simulink library "cyclopsLib"  (R2020a)
settings: Solver=VariableStepAuto  StartTime=0.0  StopTime=10.0  RelTol=1e-3
values from neighbouring files (symbols this model uses):
  agc_delay_lag = 32    [rev0BB_setup.m]
  agc_detector_coef = ones(1,agc_detector_taps)./agc_detector_taps    [rev0BB_setup.m]
  agc_sat_low = -agcSaturation    (= -12)    [rev0BB_setup.m]
  agc_sat_up = agcSaturation    (= 12)    [rev0BB_setup.m]
  agcDesired = 0    [rev0BB_setup.m]
  agcExpDomain = agcSaturation    (= 12)    [rev0BB_setup.m]
  agcExpResolution = 2^-3    (= 0.125)    [rev0BB_setup.m]
  agcPwrAvgNum = 128    [rev0BB_setup.m]
  agcSettleThresh = 0.65    [rev0BB_setup.m]
  agcStep = 2^-8    (= 0.00390625)    [rev0BB_setup.m]
  atanDomain = 5    [rev0BB_setup.m]
  atanResolution = 2^-9    (= 0.001953125)    [rev0BB_setup.m]
  bitsPerSymbolHeader = log2(radixHeader)    [rev0BB_setup.m]
  bitsPerSymbolMax = log2(radixMax)    [rev0BB_setup.m]
  cefEarlyWarning = 256    [rev0BB_setup.m]
  cefLen = length(x_CEF)    [rev0BB_setup.m]
  coarseCFOAdaptDelay = 1    [rev0BB_setup.m]
  cr_i = 0.020    (= 0.02)    [rev0BB_setup.m]
  cr_i_preamp = 2^-9    (= 0.001953125)    [rev0BB_setup.m]
  cr_int1_sat_low = -cr_integrator1_saturation    (= -0.6)    [rev0BB_setup.m]
  cr_int1_sat_up = cr_integrator1_saturation    (= 0.6)    [rev0BB_setup.m]
  cr_integrator1_decay = 1    [rev0BB_setup.m]
  cr_integrator1_saturation = 0.6    [rev0BB_setup.m]
  cr_mult_pipeline = 1    [rev0BB_setup.m]
  cr_p = 0.015    [rev0BB_setup.m]
  cr_sat2_low = -cr_saturation2    (= -0.6)    [rev0BB_setup.m]
  cr_sat2_up = cr_saturation2    (= 0.6)    [rev0BB_setup.m]
  cr_smooth_num = (1/cr_smooth_samples).*ones(1, cr_smooth_samples)    [rev0BB_setup.m]
  D_32 = [ 1,  4,  8,  2, 16]    [golay.m]    (also in rev0BB_setup.m)
  dataLenSymbols = header_len_bytes*8/bitsPerSymbolHeader + frame_len_bytes*8/bitsPerSymbol    [rev0BB_setup.m]
  delayToOutputFromDataFSM = lmsEqDepth/2-1 + regular_pipeline*9 + cr_mult_pipeline*4    (= 31)    [rev0BB_setup.m]
  enableTRFreqCorrection = true    [rev0BB_setup.m]
  expDomain = 3.3    [rev0BB_setup.m]
  expResolution = 2^-5    (= 0.03125)    [rev0BB_setup.m]
  expTol = .1    (= 0.1)    [rev0BB_setup.m]
  forceSlowRxStrobed = false    [rev0BB_setup.m]
  frac_lut_domain_cr = 64    [rev0BB_setup.m]
  frac_lut_range_max_coarse_cfo = 127    [rev0BB_setup.m]
  frac_lut_range_max_cr = 127    [rev0BB_setup.m]
  frac_lut_range_min_coarse_cfo = -frac_lut_range_max_coarse_cfo    (= -127)    [rev0BB_setup.m]
  frac_lut_range_min_cr = -frac_lut_range_max_cr    (= -127)    [rev0BB_setup.m]
  frac_lut_table_breaks_coarse_cfo = -frac_lut_domain_coarse_cfo:frac_lut_res_coarse_cfo:(frac_lut_domain_coarse_cfo-1)    [rev0BB_setup.m]
  frac_lut_table_breaks_cr = -frac_lut_domain_cr:frac_lut_res_cr:(frac_lut_domain_cr-1)    [rev0BB_setup.m]
  frac_lut_table_data_coarse_cfo = 1./frac_lut_table_breaks_coarse_cfo    [rev0BB_setup.m]
  frac_lut_table_data_cr = 1./frac_lut_table_breaks_cr    [rev0BB_setup.m]
  golay_type = 32    [rev0BB_setup.m]
  header_len_bytes = 8    [rev0BB_setup.m]
  lmsEqDepth = 38    [rev0BB_setup.m]
  lmsStep_init = 0.012    [rev0BB_setup.m]
  lmsStep_meta = (lmsStep_final - lmsStep_init)/cefLen    [rev0BB_setup.m]
  lnDomain = 16    [rev0BB_setup.m]
  lnResolution = 2^-3    (= 0.125)    [rev0BB_setup.m]
  minSTFPeaks = 3    [rev0BB_setup.m]
  mod_scheme_len_bytes = 1    [rev0BB_setup.m]
  modBPS = [1, 2, 4]    [rev0BB_setup.m]
  modKeys = [0, 1, 2]    [rev0BB_setup.m]
  mult_pipeline = 1    [rev0BB_setup.m]
  overSample = 4    [berCurve.m]    (also in rev0BB_setup.m)
  overSamplePer = 1/overSampleFreq    (= 1.25e-08)    [rev0BB_setup.m]
  qam16_demod_scale_factor = qam16_hdl_distance/qam16_power_normalized_distance    [rev0BB_setup.m]
  rcRxFilt = rcSqrtFilt    [rev0BB_setup.m]
  rcTxFilt = rcSqrtFilt    [rev0BB_setup.m]
  regular_pipeline = 1    [rev0BB_setup.m]
  rx_gain = 1    [rev0BB_setup.m]
  rx_gain_i = 1    [rev0BB_setup.m]
  rx_gain_q = 1    [rev0BB_setup.m]
  RxFeedbackPipelining = 128*3    (= 384)    [rev0BB_setup.m]
  stfLen = length(x_STF)    [rev0BB_setup.m]
  timing_differentiator_grpDelay_roundUp = ceil((timing_differentiator_len)/2)    [rev0BB_setup.m]
  timing_integrator1_decay = 0.999    [rev0BB_setup.m]
  timing_p = -1/2^2 -1/2^3    (= -0.375)    [rev0BB_setup.m]
  timing_tolerance = 4    [rev0BB_setup.m]
  timingRecoveryDoneSamplesEarly = 1    [rev0BB_setup.m]
  timingRecoveryDoneSamplesEarlyExtraDelay = -timingRecoveryDoneSamplesEarly+1    (= 0)    [rev0BB_setup.m]
  tr_int1_sat_low = -timing_integrate1_saturate    (= -0.0025)    [rev0BB_setup.m]
  tr_int1_sat_up = timing_integrate1_saturate    (= 0.0025)    [rev0BB_setup.m]
  tr_sat2_low = -timing_saturate2    (= -0.005)    [rev0BB_setup.m]
  tr_sat2_up = timing_saturate2    (= 0.005)    [rev0BB_setup.m]
  trigger = 0.40    (= 0.4)    [rev0BB_setup.m]
  trigger_tolerance = 0.35    [rev0BB_setup.m]
  W_32 = [-1,  1, -1,  1, -1]    [golay.m]    (also in rev0BB_setup.m)
  x_STFRepCount = nSpectrum_STFRepCount_short    (= 60)    [rev0BB_setup.m]
undefined symbols (not defined in the file or in its folder): agc_on, cr_integrator2_saturation, Fast_Rx_Partition, Fast_Slim_Rx_Partition, Feedback_Pipeline, freeze_en_agc, freeze_en_cr_int1, freeze_en_cr_int2, freeze_en_cr_phase, freeze_en_tr_int1, freeze_en_tr_int2, freeze_en_tr_phase, freeze_on_cef_done, freeze_on_stf_done, freeze_on_valid, i, post_cr_i_offset, post_cr_q_offset, rx_offset_correction_i, rx_offset_correction_q, Slow_Rx_Partition, timing_i, timing_i_pre_scale
libraries: simulink x62, helperLib x48, golayLib x15, commdigbbndpm3 x8, commdigbbndam3 x4, commfilt2 x3, hdlsllib x2, dspfdesign x1, simulink_need_slupdate x1, dspsigops x1, dsphdlsigops x1, $bdroot x1
(part 4 of 5)

== system cyclopsLib/cyclops_rx_combined/slow_rx_encapsulated/slow_rx/slow_rx_baseband_outer/slow_rx_baseband_enabled/slow_rx_baseband/header_parse_ack_decision ==
  note: min frame length of 2 symbols
  crc_decision : Inport
  data : Inport  Port=2
  valid : Inport  Port=3
  Data Type Conversion{4..7} (4 alike) : DataTypeConversion  Commented=on
  Delay2 : Delay  DelayLength=1  InitialCondition=0
  Display2 : Display  Commented=on
  Terminator{1..11} (11 alike) : Terminator
  Vector Concatenate1 : Concatenate  Commented=on  NumInputs=4
  header_parse_ack : Stateflow chart  TreatAsAtomicUnit=on
  majority : Subsystem
  mod_type_valid : Outport  VectorParamsAs1DForOutWhenUnconnected=off
  mod_type : Outport  Port=2  VectorParamsAs1DForOutWhenUnconnected=off
  payload_early : Outport  Port=3  VectorParamsAs1DForOutWhenUnconnected=off
  payload : Outport  Port=4  VectorParamsAs1DForOutWhenUnconnected=off
  wires:
  majority/1(Out1) -> mod_type/1
  header_parse_ack/7(mod_type) -> majority/1(In1)
  Data Type Conversion4/1 -> Vector Concatenate1/1
  Data Type Conversion5/1 -> Vector Concatenate1/2
  Data Type Conversion7/1 -> Vector Concatenate1/4
  Data Type Conversion6/1 -> Vector Concatenate1/3
  header_parse_ack/8(type) -> Terminator9/1, Data Type Conversion4/1
  header_parse_ack/6(done_parsing) -> Terminator7/1
  valid/1 -> header_parse_ack/2(valid)
  header_parse_ack/4(dst_valid) -> Terminator5/1
  header_parse_ack/5(len_valid) -> Terminator6/1
  header_parse_ack/3(src_valid) -> Terminator4/1
  data/1 -> header_parse_ack/1(data)
  crc_decision/1 -> Delay2/1
  header_parse_ack/9(src) -> Terminator8/1, Data Type Conversion5/1
  Delay2/1 -> header_parse_ack/3(rst)
  Vector Concatenate1/1 -> Display2/1
  header_parse_ack/10(dst) -> Data Type Conversion6/1, Terminator2/1
  header_parse_ack/11(len) -> Terminator1/1, Data Type Conversion7/1
  header_parse_ack/2(type_valid) -> Terminator3/1
  header_parse_ack/1(mod_type_valid) -> mod_type_valid/1
  header_parse_ack/13(payload_early) -> payload_early/1
  header_parse_ack/12(payload) -> payload/1
  header_parse_ack/14(net_id_valid) -> Terminator10/1
  header_parse_ack/15(net_id) -> Terminator11/1

== system cyclopsLib/cyclops_rx_combined/slow_rx_encapsulated/slow_rx/slow_rx_baseband_outer/slow_rx_baseband_enabled/slow_rx_baseband/mod_data_buffer ==
  data : Inport
  header : Inport  Port=2
  payload : Inport  Port=3
  last_in : Inport  Port=4
  bitsPerSymbolPayload : Inport  Port=5
  rst : Inport  Port=6
  header_parse_and_buffer : Stateflow chart  TreatAsAtomicUnit=on
  packed_data : Outport  VectorParamsAs1DForOutWhenUnconnected=off
  valid : Outport  Port=2  VectorParamsAs1DForOutWhenUnconnected=off
  last_out : Outport  Port=3  VectorParamsAs1DForOutWhenUnconnected=off
  decoding : Outport  Port=4  VectorParamsAs1DForOutWhenUnconnected=off
  err : Outport  Port=5  VectorParamsAs1DForOutWhenUnconnected=off
  wires:
  data/1 -> header_parse_and_buffer/4(data)
  header/1 -> header_parse_and_buffer/2(header)
  header_parse_and_buffer/2(packed_data) -> packed_data/1
  header_parse_and_buffer/3(valid) -> valid/1
  header_parse_and_buffer/1(last_out) -> last_out/1
  payload/1 -> header_parse_and_buffer/5(payload)
  last_in/1 -> header_parse_and_buffer/1(last_in)
  bitsPerSymbolPayload/1 -> header_parse_and_buffer/3(bitsPerSymbolMod)
  rst/1 -> header_parse_and_buffer/6(rst)
  header_parse_and_buffer/4(decoding) -> decoding/1
  header_parse_and_buffer/5(err) -> err/1

== system cyclopsLib/cyclops_rx_combined/slow_rx_encapsulated/slow_rx/slow_rx_baseband_outer/slow_rx_baseband_enabled/slow_rx_baseband/nco ==
  incr : Inport
  Data Type Conversion3 : DataTypeConversion  OutDataTypeStr=int32
  Display : Display  Commented=on
  Display1 : Display  Commented=on
  NCO : dspsigops/NCO  AccIncSrc=Input port  AccInc=100  PhaseOffsetSrc=Specify via dialog  PhaseOffset=0  AccumWL=16  HasDither=off  DitherWL=4  PNgeneratorLength=19  HasPhaseQuantizer=on  TableDepth=12  HasOutputPhaseError=off  Formula=Complex exponential  DataType=single  OutputWL=18  OutputFL=13  CompMethod=Table lookup (no interpolation)  SampleTime=1  SamplesPerFrame=1  OutputFrames=off
      settings: SourceProductBaseCode=DS
  NCO HDL Optimized : dsphdlsigops/NCO HDL Optimized  Commented=on  PhaseIncrementSource=Input port  PhaseIncrement=100  PhaseOffsetSource=Property  PhaseOffset=0  DitherSource=None  NumDitherBits=4  SamplesPerFrame=1  LUTCompress=on  ResetAction=off  Waveform=Complex exponential  PhasePort=on  SimulateUsing=Code generation  AccumulatorWL=22  PhaseQuantization=on  NumQuantizerAccumulatorBits=20  OutputDataType=Binary point scaling  OutputWL=18  OutputFL=13
      settings: SourceProductBaseCode=DS
  Signal Specification : SignalSpecification  Commented=on  Dimensions=1
  Terminator1 : Terminator  Commented=on
  nco_phase : Scope  Commented=on
  incr_int : Outport  VectorParamsAs1DForOutWhenUnconnected=off
  complex_sin : Outport  Port=2  VectorParamsAs1DForOutWhenUnconnected=off
  wires:
  Data Type Conversion3/1 -> Display1/1, NCO/1, incr_int/1, Signal Specification/1
  NCO/1 -> complex_sin/1
  incr/1 -> Display/1, Data Type Conversion3/1
  NCO HDL Optimized/3 -> Terminator1/1
  NCO HDL Optimized/2 -> nco_phase/1

== system cyclopsLib/cyclops_rx_combined/slow_rx_encapsulated/slow_rx/slow_rx_baseband_outer/slow_rx_baseband_enabled/slow_rx_baseband/preamble_data_ctrl ==
  stfStart : Inport
  cefStart : Inport  Port=2
  Data Type Conversion : DataTypeConversion  OutDataTypeStr=boolean
  Terminator : Terminator
  Terminator1 : Terminator
  cef_eq_fsm : Stateflow chart  TreatAsAtomicUnit=on
  data_control : Stateflow chart  TreatAsAtomicUnit=on
  dataValid : Outport  VectorParamsAs1DForOutWhenUnconnected=off
  cefSymb : Outport  Port=2  VectorParamsAs1DForOutWhenUnconnected=off
  dataLast : Outport  Port=3  VectorParamsAs1DForOutWhenUnconnected=off
  err : Outport  Port=4  VectorParamsAs1DForOutWhenUnconnected=off
  stf : Outport  Port=5  VectorParamsAs1DForOutWhenUnconnected=off
  cef : Outport  Port=6  VectorParamsAs1DForOutWhenUnconnected=off
  cefCount : Outport  Port=7  VectorParamsAs1DForOutWhenUnconnected=off
  preamble_done : Outport  Port=8  VectorParamsAs1DForOutWhenUnconnected=off
  cefEarly : Outport  Port=9  VectorParamsAs1DForOutWhenUnconnected=off
  ack : Outport  Port=10  VectorParamsAs1DForOutWhenUnconnected=off
  ack_done : Outport  Port=11  VectorParamsAs1DForOutWhenUnconnected=off
  ack_dst : Outport  Port=12  VectorParamsAs1DForOutWhenUnconnected=off
  ack_trigger : Outport  Port=13  VectorParamsAs1DForOutWhenUnconnected=off
  dataLast_early : Outport  Port=14  VectorParamsAs1DForOutWhenUnconnected=off
  wires:
  data_control/3(earlyLast) -> dataLast_early/1
  cefStart/1 -> cef_eq_fsm/2(cef_start)
  stfStart/1 -> cef_eq_fsm/1(stf_start)
  cef_eq_fsm/1(data) -> Data Type Conversion/1
  cef_eq_fsm/3(cefSymb) -> cefSymb/1
  cef_eq_fsm/6(cefCount) -> cefCount/1
  cef_eq_fsm/7(cef_early) -> cefEarly/1
  data_control/1(valid) -> dataValid/1
  cef_eq_fsm/2(err) -> err/1
  cef_eq_fsm/4(stf) -> stf/1
  cef_eq_fsm/5(cef) -> cef/1
  data_control/2(last) -> dataLast/1
  cef_eq_fsm/8(waiting) -> Terminator/1
  cef_eq_fsm/10(ack) -> ack/1
  cef_eq_fsm/9(ack_done) -> ack_done/1
  cef_eq_fsm/11(ack_dst) -> ack_dst/1
  cef_eq_fsm/12(ack_count) -> Terminator1/1
  cef_eq_fsm/13(ack_trigger) -> ack_trigger/1
  Data Type Conversion/1 -> preamble_done/1, data_control/1(preamble_done)

== system cyclopsLib/cyclops_rx_combined/slow_rx_encapsulated/slow_rx/slow_rx_baseband_outer/slow_rx_baseband_enabled/slow_rx_baseband/CoarseCFO_est/atan ==
  note: 5 delays
  note: Special case for undefined ouput of atan2.
      | To produce an unbiased ouput, this should be 0.
  imag_y : Inport
  real_x : Inport  Port=2
  Compare To Constant2 : simulink/Logic and Bit Operations/Compare To Constant  relop=>=  const=0  OutDataTypeStr=boolean
  Compare To Constant3 : simulink/Logic and Bit Operations/Compare To Constant  relop===  const=0  OutDataTypeStr=boolean
  Compare To Constant4 : simulink/Logic and Bit Operations/Compare To Constant  relop===  const=0  OutDataTypeStr=boolean
  Constant2 : Constant  Value=0  OutDataTypeStr=Inherit: Inherit via back propagation  SampleTime=-1
  Constant3 : Constant  Value=-pi/2  OutDataTypeStr=Inherit: Inherit via back propagation  SampleTime=-1
  Constant4 : Constant  Value=pi/2  OutDataTypeStr=Inherit: Inherit via back propagation  SampleTime=-1
  Logical Operator : Logic  AllPortsSameDT=off  OutDataTypeStr=boolean
  Logical Operator1 : Logic  AllPortsSameDT=off  OutDataTypeStr=boolean
  Switch3 : Switch  Criteria=u2 ~= 0  OutDataTypeStr=Inherit: Inherit via back propagation
  Switch4 : Switch  Criteria=u2 ~= 0  OutDataTypeStr=Inherit: Inherit via back propagation
  Switch5 : Switch  Criteria=u2 ~= 0  OutDataTypeStr=Inherit: Inherit via back propagation
  bound_atan : Subsystem  AncestorBlock=helperLib/bound_atan
  inv : Subsystem
  mult_delay_match : Delay  DelayLength=cr_mult_pipeline*2+regular_pipeline*2
  pipeline_delay{,1..3} (4 alike) : Delay  DelayLength=regular_pipeline
  pipeline_delay_match2 : Delay  DelayLength=cr_mult_pipeline*5+regular_pipeline*7
  pipeline_delay_match3 : Delay  DelayLength=cr_mult_pipeline*5+regular_pipeline*7
  pipeline_delay_match4 : Delay  DelayLength=cr_mult_pipeline*5+regular_pipeline*7
  pipelined_mult : helperLib/pipelined_mult  d=cr_mult_pipeline
  Out1 : Outport  VectorParamsAs1DForOutWhenUnconnected=off
  wires:
  pipeline_delay1/1 -> bound_atan/1(In1)
  imag_y/1 -> Compare To Constant4/1, Compare To Constant2/1, mult_delay_match/1
  mult_delay_match/1 -> pipeline_delay2/1
  bound_atan/1(Out1) -> pipeline_delay/1
  pipelined_mult/1 -> pipeline_delay1/1
  pipeline_delay2/1 -> pipelined_mult/1
  pipeline_delay3/1 -> pipelined_mult/2
  Compare To Constant4/1 -> Logical Operator/1
  Logical Operator/1 -> pipeline_delay_match2/1
  pipeline_delay_match2/1 -> Switch3/2
  real_x/1 -> inv/1(In), Compare To Constant3/1
  inv/1(Out) -> pipeline_delay3/1
  Switch4/1 -> Switch5/3
  Constant3/1 -> Switch4/1
  Constant4/1 -> Switch5/1
  Switch5/1 -> Switch3/3
  Constant2/1 -> Switch3/1
  Compare To Constant3/1 -> Logical Operator1/2, pipeline_delay_match4/1, Logical Operator/2
  Logical Operator1/1 -> pipeline_delay_match3/1
  pipeline_delay_match3/1 -> Switch5/2
  pipeline_delay_match4/1 -> Switch4/2
  Compare To Constant2/1 -> Logical Operator1/1
  pipeline_delay/1 -> Switch4/3
  Switch3/1 -> Out1/1

== system cyclopsLib/cyclops_rx_combined/slow_rx_encapsulated/slow_rx/slow_rx_baseband_outer/slow_rx_baseband_enabled/slow_rx_baseband/CoarseCFO_est/complex_mult_pipelined1 ==
  In1 : Inport
  In2 : Inport  Port=2
  Add1 : Sum  OutDataTypeStr=Inherit: Same as first input
  Add2 : Sum  OutDataTypeStr=Inherit: Same as first input
  Complex to Real-Imag3 : ComplexToRealImag
  Complex to Real-Imag4 : ComplexToRealImag
  Real-Imag to Complex2 : RealImagToComplex
  mult_delay_match3 : Delay  DelayLength=cr_mult_pipeline
  mult_delay_match4 : Delay  DelayLength=cr_mult_pipeline
  mult_delay_match5 : Delay  DelayLength=cr_mult_pipeline
  pipeline_delay{1..3,6} (4 alike) : Delay  DelayLength=regular_pipeline
  pipelined_gain : helperLib/pipelined_gain  g=-1  d=cr_mult_pipeline
  pipelined_mult{,1..3} (4 alike) : helperLib/pipelined_mult  d=cr_mult_pipeline
  Out1 : Outport  VectorParamsAs1DForOutWhenUnconnected=off
  wires:
  pipelined_gain/1 -> Add1/2
  pipelined_mult3/1 -> mult_delay_match5/1
  pipelined_mult2/1 -> mult_delay_match4/1
  pipelined_mult1/1 -> pipelined_gain/1
  pipelined_mult/1 -> mult_delay_match3/1
  Complex to Real-Imag4/1 -> pipelined_mult/2, pipelined_mult3/2
  Complex to Real-Imag3/2 -> pipelined_mult1/1, pipelined_mult3/1
  Complex to Real-Imag4/2 -> pipelined_mult2/2, pipelined_mult1/2
  Complex to Real-Imag3/1 -> pipelined_mult2/1, pipelined_mult/1
  pipeline_delay3/1 -> Complex to Real-Imag4/1
  pipeline_delay2/1 -> Complex to Real-Imag3/1
  Add2/1 -> pipeline_delay6/1
  Add1/1 -> pipeline_delay1/1
  In1/1 -> pipeline_delay2/1
  mult_delay_match5/1 -> Add2/2
  pipeline_delay1/1 -> Real-Imag to Complex2/1
  In2/1 -> pipeline_delay3/1
  pipeline_delay6/1 -> Real-Imag to Complex2/2
  Real-Imag to Complex2/1 -> Out1/1
  mult_delay_match3/1 -> Add1/1
  mult_delay_match4/1 -> Add2/1

== system cyclopsLib/cyclops_rx_combined/slow_rx_encapsulated/slow_rx/slow_rx_baseband_outer/slow_rx_baseband_enabled/slow_rx_baseband/EQ/lms ==
  in : Inport
  expected : Inport  Port=2
  reset : Inport  Port=3
  adapt : Inport  Port=4
  step : Inport  Port=5
  Constant : Constant  Value=complex(cat(1,zeros(lmsEqDepth/2-1,1), [1], zeros(lmsEqDepth/2,1)))  OutDataTypeStr=Inherit: Inherit via back propagation  SampleTime=-1
  Data Type Conversion : DataTypeConversion  OutDataTypeStr=single
  Data Type Conversion1 : DataTypeConversion  OutDataTypeStr=single
  Data Type Conversion2 : DataTypeConversion  OutDataTypeStr=single
  Delay : Delay  DelayLength=1
  Delay3 : Delay  DelayLength=lmsEqDepth/2-1  InitialCondition=0
  Discrete FIR Filter : DiscreteFir  CoefSource=Input port  FilterStructure=Direct form transposed  OutDataTypeStr=Inherit: Same as input
      settings: InputPortMap=u0,u1
  Display : Display  Commented=on
  Product : Product  OutDataTypeStr=Inherit: Same as first input
  Product1 : Product  OutDataTypeStr=Inherit: Same as first input
  Sum : Sum  Inputs=|+-  OutDataTypeStr=Inherit: Same as first input
  Sum1 : Sum  Inputs=|++  OutDataTypeStr=Inherit: Same as first input
  Switch : Switch  Criteria=u2 > Threshold
  Switch1 : Switch  Criteria=u2 > Threshold
  Tapped Delay : simulink/Discrete/Tapped Delay  vinit=0.0  samptime=-1  NumDelays=lmsEqDepth-1  DelayOrder=Newest  includeCurrent=off
  Unit Delay Resettable : simulink_need_slupdate/Unit Delay Resettable  Commented=on  vinit=complex(cat(1,zeros(lmsEqDepth/2-1,1), [1], zeros(lmsEqDepth/2,1)))  tsamp=-1
      settings: SourceProductBaseCode=SL
  Vector Concatenate : Concatenate
  complex_conj : helperLib/complex_conj  SystemSampleTime=-1  Latency=0  AutoFrameSizeCalculation=off
  pipeline_delay{1,3..6} (5 alike) : Delay  DelayLength=regular_pipeline
  out : Outport  VectorParamsAs1DForOutWhenUnconnected=off
  err : Outport  Port=2  VectorParamsAs1DForOutWhenUnconnected=off
  wires:
  Tapped Delay/1 -> Vector Concatenate/2
  Data Type Conversion2/1 -> pipeline_delay6/1
  complex_conj/1 -> Tapped Delay/1, Vector Concatenate/1
  Sum1/1 -> Switch/1
  Data Type Conversion1/1 -> pipeline_delay1/1
  Data Type Conversion/1 -> Delay3/1
  step/1 -> pipeline_delay3/1
  Delay3/1 -> pipeline_delay4/1
  adapt/1 -> Switch/2
  pipeline_delay1/1 -> complex_conj/1, Discrete FIR Filter/1
  Delay/1 -> Sum1/1, Display/1, Switch/3, Discrete FIR Filter/2
  reset/1 -> Switch1/2
  expected/1 -> Data Type Conversion/1
  in/1 -> Data Type Conversion1/1
  pipeline_delay5/1 -> err/1
  pipeline_delay6/1 -> out/1
  Sum/1 -> Product/1, pipeline_delay5/1
  pipeline_delay3/1 -> Product/2
  Product/1 -> Product1/1
  Vector Concatenate/1 -> Product1/2
  pipeline_delay4/1 -> Sum/1
  Discrete FIR Filter/1 -> Sum/2, Data Type Conversion2/1
  Product1/1 -> Sum1/2
  Switch/1 -> Switch1/3
  Switch1/1 -> Delay/1
  Constant/1 -> Switch1/1

== system cyclopsLib/cyclops_rx_combined/slow_rx_encapsulated/slow_rx/slow_rx_baseband_outer/slow_rx_baseband_enabled/slow_rx_baseband/FineCarrierRecovery/Est_Phase ==
  In1 : Inport
  ModMode : Inport  Port=2
  Atan2 : Trigonometry  Operator=atan2
  Complex to Real-Imag : ComplexToRealImag
  Complex to Real-Imag1 : ComplexToRealImag
  Data Type Conversion : DataTypeConversion  OutDataTypeStr=single
  Gain : Gain  Gain=-1  OutDataTypeStr=Inherit: Same as input
  Real-Imag to Complex1 : RealImagToComplex
  atan2 : Subsystem  Commented=on  AncestorBlock=helperLib/atan2
  complex_mult_pipelined1 : Subsystem  AncestorBlock=helperLib/complex_mult_pipelined
  find_nearest : Subsystem
  mult_delay5 : Delay  DelayLength=cr_mult_pipeline
  mult_delay_match : Delay  DelayLength=cr_mult_pipeline
  mult_delay_match2 : Delay  DelayLength=cr_mult_pipeline
  pipeline_delay2 : Delay  DelayLength=regular_pipeline
  phase_offset : Outport  VectorParamsAs1DForOutWhenUnconnected=off
  wires:
  mult_delay_match2/1 -> complex_mult_pipelined1/1(In1)
  find_nearest/1(Out1) -> mult_delay_match2/1
  Data Type Conversion/1 -> Complex to Real-Imag/1, find_nearest/1(In1)
  Atan2/1 -> pipeline_delay2/1
  Complex to Real-Imag1/2 -> Atan2/1
  Complex to Real-Imag1/1 -> Atan2/2
  pipeline_delay2/1 -> phase_offset/1
  Gain/1 -> Real-Imag to Complex1/2
  mult_delay_match/1 -> Real-Imag to Complex1/1
  Real-Imag to Complex1/1 -> complex_mult_pipelined1/2(In2)
  Complex to Real-Imag/2 -> mult_delay5/1
  Complex to Real-Imag/1 -> mult_delay_match/1
  In1/1 -> Data Type Conversion/1
  mult_delay5/1 -> Gain/1
  complex_mult_pipelined1/1(Out1) -> Complex to Real-Imag1/1
  ModMode/1 -> find_nearest/2(ModMode)

== system cyclopsLib/cyclops_rx_combined/slow_rx_encapsulated/slow_rx/slow_rx_baseband_outer/slow_rx_baseband_enabled/slow_rx_baseband/FineCarrierRecovery/PostCR_IQ_Offset_Correct ==
  In : Inport
  post_cr_i_offset : Inport  Port=2
  post_cr_q_offset : Inport  Port=3
  Add : Sum  OutDataTypeStr=Inherit: Same as first input
  Add1 : Sum  OutDataTypeStr=Inherit: Same as first input
  Complex to Real-Imag1 : ComplexToRealImag
  Real-Imag to Complex1 : RealImagToComplex
  pipeline_delay : Delay  DelayLength=regular_pipeline
  pipeline_delay1 : Delay  DelayLength=regular_pipeline
  Out : Outport  VectorParamsAs1DForOutWhenUnconnected=off
  wires:
  Real-Imag to Complex1/1 -> Out/1
  Add/1 -> pipeline_delay/1
  Complex to Real-Imag1/2 -> Add1/1
  Complex to Real-Imag1/1 -> Add/1
  Add1/1 -> pipeline_delay1/1
  In/1 -> Complex to Real-Imag1/1
  post_cr_q_offset/1 -> Add1/2
  post_cr_i_offset/1 -> Add/2
  pipeline_delay/1 -> Real-Imag to Complex1/1
  pipeline_delay1/1 -> Real-Imag to Complex1/2

== system cyclopsLib/cyclops_rx_combined/slow_rx_encapsulated/slow_rx/slow_rx_baseband_outer/slow_rx_baseband_enabled/slow_rx_baseband/FineCarrierRecovery/complex_mult_pipelined ==
  In1 : Inport
  In2 : Inport  Port=2
  Add1 : Sum  OutDataTypeStr=Inherit: Same as first input
  Add2 : Sum  OutDataTypeStr=Inherit: Same as first input
  Complex to Real-Imag3 : ComplexToRealImag
  Complex to Real-Imag4 : ComplexToRealImag
  Real-Imag to Complex2 : RealImagToComplex
  mult_delay_match3 : Delay  DelayLength=cr_mult_pipeline
  mult_delay_match4 : Delay  DelayLength=cr_mult_pipeline
  mult_delay_match5 : Delay  DelayLength=cr_mult_pipeline
  pipeline_delay{1..3,6} (4 alike) : Delay  DelayLength=regular_pipeline
  pipelined_gain : helperLib/pipelined_gain  g=-1  d=cr_mult_pipeline
  pipelined_mult{,1..3} (4 alike) : helperLib/pipelined_mult  d=cr_mult_pipeline
  Out1 : Outport  VectorParamsAs1DForOutWhenUnconnected=off
  wires:
  pipelined_gain/1 -> Add1/2
  pipelined_mult3/1 -> mult_delay_match5/1
  pipelined_mult2/1 -> mult_delay_match4/1
  pipelined_mult1/1 -> pipelined_gain/1
  pipelined_mult/1 -> mult_delay_match3/1
  Complex to Real-Imag4/1 -> pipelined_mult/2, pipelined_mult3/2
  Complex to Real-Imag3/2 -> pipelined_mult1/1, pipelined_mult3/1
  Complex to Real-Imag4/2 -> pipelined_mult2/2, pipelined_mult1/2
  Complex to Real-Imag3/1 -> pipelined_mult2/1, pipelined_mult/1
  pipeline_delay3/1 -> Complex to Real-Imag4/1
  pipeline_delay2/1 -> Complex to Real-Imag3/1
  Add2/1 -> pipeline_delay6/1
  Add1/1 -> pipeline_delay1/1
  In1/1 -> pipeline_delay2/1
  mult_delay_match5/1 -> Add2/2
  pipeline_delay1/1 -> Real-Imag to Complex2/1
  In2/1 -> pipeline_delay3/1
  pipeline_delay6/1 -> Real-Imag to Complex2/2
  Real-Imag to Complex2/1 -> Out1/1
  mult_delay_match3/1 -> Add1/1
  mult_delay_match4/1 -> Add2/1

== system cyclopsLib/cyclops_rx_combined/slow_rx_encapsulated/slow_rx/slow_rx_baseband_outer/slow_rx_baseband_enabled/slow_rx_baseband/FineCarrierRecovery/overflow_protect ==
  note: Synthesizer
  note: This fixes overflow problem with LUT.  This keeps the
      | signal from -pi to pi plus some hystoresis if the LUT's
      | domain is slightly larger than -pi to pi
  In1 : Inport
  Compare To Constant2 : simulink/Logic and Bit Operations/Compare To Constant  relop=>=  const=expDomain-expTol  OutDataTypeStr=boolean
  Compare To Constant3 : simulink/Logic and Bit Operations/Compare To Constant  relop=<=  const=-expDomain+expTol  OutDataTypeStr=boolean
  Constant1 : Constant  Value=2*pi  OutDataTypeStr=Inherit: Inherit via back propagation  SampleTime=-1
  Constant2 : Constant  Value=0  OutDataTypeStr=Inherit: Inherit via back propagation  SampleTime=-1
  Sum4 : Sum  Inputs=|+-  OutDataTypeStr=Inherit: Same as first input
  Sum5 : Sum  Inputs=|++  OutDataTypeStr=Inherit: Same as first input
  Switch : Switch  Criteria=u2 ~= 0  OutDataTypeStr=Inherit: Inherit via back propagation
  Switch1 : Switch  Criteria=u2 ~= 0  OutDataTypeStr=Inherit: Inherit via back propagation
  Out1 : Outport  VectorParamsAs1DForOutWhenUnconnected=off
  wires:
  Sum4/1 -> Out1/1
  Compare To Constant3/1 -> Switch/2
  Compare To Constant2/1 -> Switch1/2
  Constant1/1 -> Switch/1, Switch1/1
  Constant2/1 -> Switch1/3, Switch/3
  Switch/1 -> Sum5/2
  Sum5/1 -> Sum4/1
  Switch1/1 -> Sum4/2
  In1/1 -> Sum5/1, Compare To Constant3/1, Compare To Constant2/1

== system cyclopsLib/cyclops_rx_combined/slow_rx_encapsulated/slow_rx/slow_rx_baseband_outer/slow_rx_baseband_enabled/slow_rx_baseband/FineCarrierRecovery/scale_and_loop ==
  phase_offset : Inport
  cr_i_preamp : Inport  Port=2
  cr_p : Inport  Port=3
  cr_i : Inport  Port=4
  cr_integrator1_decay : Inport  Port=5
  cr_int1_sat_up : Inport  Port=6
  cr_int1_sat_low : Inport  Port=7
  cr_sat2_up : Inport  Port=8
  cr_sat2_low : Inport  Port=9
  cr_int1_freeze : Inport  Port=10
  reset : Inport  Port=11
  Loop Filter : Subsystem
  pipeline_delay8 : Delay  DelayLength=regular_pipeline
  correction : Outport  VectorParamsAs1DForOutWhenUnconnected=off
  wires:
  Loop Filter/1(Out) -> pipeline_delay8/1
  phase_offset/1 -> Loop Filter/1(PhaseOffset)
  pipeline_delay8/1 -> correction/1
  cr_i_preamp/1 -> Loop Filter/2(cr_i_preamp)
  cr_p/1 -> Loop Filter/3(cr_p)
  cr_i/1 -> Loop Filter/4(cr_i)
  cr_integrator1_decay/1 -> Loop Filter/5(cr_integrator1_decay)
  cr_sat2_low/1 -> Loop Filter/9(cr_sat2_low)
  cr_sat2_up/1 -> Loop Filter/8(cr_sat2_up)
  cr_int1_sat_low/1 -> Loop Filter/7(cr_int1_sat_low)
  cr_int1_sat_up/1 -> Loop Filter/6(cr_int1_sat_up)
  cr_int1_freeze/1 -> Loop Filter/10(int1_freeze)
  reset/1 -> Loop Filter/11(reset)

== system cyclopsLib/cyclops_rx_combined/slow_rx_encapsulated/slow_rx/slow_rx_baseband_outer/slow_rx_baseband_enabled/slow_rx_baseband/FineCarrierRecovery/shift180 ==
  note: Todo: propogate this conversion back
  In1 : Inport
  shift180 : Inport  Port=2
  Constant8 : Constant  Value=0  OutDataTypeStr=Inherit: Inherit via back propagation  SampleTime=-1
  Constant9 : Constant  Value=pi  OutDataTypeStr=Inherit: Inherit via back propagation  SampleTime=-1
  Sum6 : Sum  Inputs=|++  OutDataTypeStr=Inherit: Same as first input
  Switch6 : Switch  Criteria=u2 ~= 0  OutDataTypeStr=Inherit: Inherit via back propagation
  pipeline_delay_match1 : Delay  DelayLength=regular_pipeline
  Out1 : Outport  VectorParamsAs1DForOutWhenUnconnected=off
  wires:
  In1/1 -> Sum6/1
  shift180/1 -> pipeline_delay_match1/1
  Constant9/1 -> Switch6/1
  Constant8/1 -> Switch6/3
  Sum6/1 -> Out1/1
  Switch6/1 -> Sum6/2
  pipeline_delay_match1/1 -> Switch6/2

== system cyclopsLib/cyclops_rx_combined/slow_rx_encapsulated/slow_rx/slow_rx_baseband_outer/slow_rx_baseband_enabled/slow_rx_baseband/header_parse_ack_decision/majority ==
  In1 : Inport
  Bit Shift1 : hdlsllib/Logic and Bit Operations/Bit Shift  mode=Shift Right Logical  N=2
  Bit Shift2 : hdlsllib/Logic and Bit Operations/Bit Shift  mode=Shift Right Logical  N=4
  Bitwise AND : simulink/Logic and Bit Operations/Bitwise Operator  logicop=AND  UseBitMask=on  BitMask=bin2dec('00000011')  BitMaskRealWorld=Stored Integer
  Bitwise AND1 : simulink/Logic and Bit Operations/Bitwise Operator  logicop=AND  UseBitMask=on  BitMask=bin2dec('00000011')  BitMaskRealWorld=Stored Integer
  Bitwise AND2 : simulink/Logic and Bit Operations/Bitwise Operator  logicop=AND  UseBitMask=on  BitMask=bin2dec('00000011')  BitMaskRealWorld=Stored Integer
  Bitwise AND3 : simulink/Logic and Bit Operations/Bitwise Operator  logicop=AND  UseBitMask=off  NumInputPorts=2  BitMask=bin2dec('11011001')  BitMaskRealWorld=Stored Integer
  Bitwise AND4 : simulink/Logic and Bit Operations/Bitwise Operator  logicop=AND  UseBitMask=off  NumInputPorts=2  BitMask=bin2dec('11011001')  BitMaskRealWorld=Stored Integer
  Bitwise AND5 : simulink/Logic and Bit Operations/Bitwise Operator  logicop=AND  UseBitMask=off  NumInputPorts=2  BitMask=bin2dec('11011001')  BitMaskRealWorld=Stored Integer
  Bitwise OR : simulink/Logic and Bit Operations/Bitwise Operator  logicop=OR  UseBitMask=off  NumInputPorts=3  BitMask=bin2dec('11011001')  BitMaskRealWorld=Stored Integer
  Out1 : Outport
  wires:
  Bitwise AND2/1 -> Bitwise AND4/2, Bitwise AND5/2
  In1/1 -> Bitwise AND/1, Bit Shift1/1, Bit Shift2/1
  Bitwise AND4/1 -> Bitwise OR/2
  Bitwise AND1/1 -> Bitwise AND3/2, Bitwise AND4/1
  Bitwise AND/1 -> Bitwise AND3/1, Bitwise AND5/1
  Bitwise AND3/1 -> Bitwise OR/1
  Bit Shift2/1 -> Bitwise AND2/1
  Bit Shift1/1 -> Bitwise AND1/1
  Bitwise AND5/1 -> Bitwise OR/3
  Bitwise OR/1 -> Out1/1

== system cyclopsLib/cyclops_rx_combined/slow_rx_encapsulated/slow_rx/slow_rx_baseband_outer/slow_rx_baseband_enabled/slow_rx_baseband/CoarseCFO_est/atan/bound_atan ==
  note: Bound Protection
  In1 : Inport
  Compare To Constant1 : simulink/Logic and Bit Operations/Compare To Constant  relop=>=  const=atanDomain  OutDataTypeStr=boolean
  Compare To Constant4 : simulink/Logic and Bit Operations/Compare To Constant  relop=<=  const=-atanDomain  OutDataTypeStr=boolean
  Constant11 : Constant  Value=0  OutDataTypeStr=Inherit: Inherit via back propagation  SampleTime=-1
  Constant3 : Constant  Value=pi/2  OutDataTypeStr=Inherit: Inherit via back propagation  SampleTime=-1
  Constant4 : Constant  Value=-pi/2  OutDataTypeStr=Inherit: Inherit via back propagation  SampleTime=-1
  Data Type Duplicate : DataTypeDuplicate
  Data Type Duplicate1 : DataTypeDuplicate
  Data Type Duplicate2 : DataTypeDuplicate
  Data Type Conversion : DataTypeConversion  OutDataTypeStr=single
  Logical Operator : Logic  Operator=OR  AllPortsSameDT=off  OutDataTypeStr=boolean
  Switch2 : Switch  Criteria=u2 ~= 0  OutDataTypeStr=Inherit: Inherit via back propagation
  Switch3 : Switch  Criteria=u2 ~= 0  OutDataTypeStr=Inherit: Inherit via back propagation
  Switch8 : Switch  Criteria=u2 ~= 0  OutDataTypeStr=Inherit: Inherit via back propagation
  atan Lookup Table : Lookup_n-D  NumberOfTableDimensions=1  BreakpointsForDimension1=[-atanDomain:atanResolution:atanDomain]  IndexSearchMethod=Evenly spaced points  Table=atan([-atanDomain:atanResolution:atanDomain])  InterpMethod=Flat  DiagnosticForOutOfRangeInput=Error  RemoveProtectionInput=on  InternalRulePriority=Speed  OutDataTypeStr=Inherit: Inherit via back propagation  RndMeth=Simplest  InputSameDT=on
  mult_delay : Delay  DelayLength=cr_mult_pipeline
  mult_delay_match : Delay  DelayLength=cr_mult_pipeline
  mult_delay_match1 : Delay  DelayLength=cr_mult_pipeline
  pipeline_delay1 : Delay  DelayLength=regular_pipeline*2
  pipeline_delay2 : Delay  DelayLength=regular_pipeline
  pipeline_delay_match : Delay  DelayLength=regular_pipeline*3
  pipeline_delay_match1 : Delay  DelayLength=regular_pipeline*3
  Out1 : Outport  VectorParamsAs1DForOutWhenUnconnected=off
  wires:
  pipeline_delay2/1 -> Data Type Duplicate2/1, Switch2/3
  mult_delay/1 -> atan Lookup Table/1
  pipeline_delay1/1 -> mult_delay/1
  mult_delay_match1/1 -> Switch3/2
  mult_delay_match/1 -> Switch2/2
  pipeline_delay_match1/1 -> mult_delay_match1/1
  pipeline_delay_match/1 -> mult_delay_match/1
  atan Lookup Table/1 -> Data Type Duplicate/2, pipeline_delay2/1
  Switch8/1 -> Data Type Conversion/1
  Constant11/1 -> Switch8/1
  Logical Operator/1 -> Switch8/2
  In1/1 -> Data Type Duplicate/1, Compare To Constant4/1, Compare To Constant1/1, Switch8/3
  Switch3/1 -> Data Type Duplicate2/2, Data Type Duplicate1/2, Out1/1
  Constant4/1 -> Switch3/1
  Switch2/1 -> Data Type Duplicate1/1, Switch3/3
  Constant3/1 -> Switch2/1
  Compare To Constant4/1 -> pipeline_delay_match1/1, Logical Operator/2
  Compare To Constant1/1 -> pipeline_delay_match/1, Logical Operator/1
  Data Type Conversion/1 -> pipeline_delay1/1

== system cyclopsLib/cyclops_rx_combined/slow_rx_encapsulated/slow_rx/slow_rx_baseband_outer/slow_rx_baseband_enabled/slow_rx_baseband/CoarseCFO_est/atan/inv ==
  note: Bound Protection
  In : Inport
  Compare To Constant1 : simulink/Logic and Bit Operations/Compare To Constant  relop=>=  const=frac_lut_domain_cr-1  OutDataTypeStr=boolean
  Compare To Constant4 : simulink/Logic and Bit Operations/Compare To Constant  relop=<=  const=-frac_lut_domain_cr  OutDataTypeStr=boolean
  Constant11 : Constant  Value=0  OutDataTypeStr=Inherit: Inherit via back propagation  SampleTime=-1
  Constant3 : Constant  Value=frac_lut_range_max_coarse_cfo  OutDataTypeStr=Inherit: Inherit via back propagation  SampleTime=-1
  Constant4 : Constant  Value=frac_lut_range_min_coarse_cfo  OutDataTypeStr=Inherit: Inherit via back propagation  SampleTime=-1
  Data Type Duplicate : DataTypeDuplicate
  Data Type Duplicate1 : DataTypeDuplicate
  Data Type Duplicate2 : DataTypeDuplicate
  Data Type Conversion : DataTypeConversion  OutDataTypeStr=single
  Logical Operator : Logic  Operator=OR  AllPortsSameDT=off  OutDataTypeStr=boolean
  Switch2 : Switch  Criteria=u2 ~= 0  OutDataTypeStr=Inherit: Inherit via back propagation
  Switch3 : Switch  Criteria=u2 ~= 0  OutDataTypeStr=Inherit: Inherit via back propagation
  Switch8 : Switch  Criteria=u2 ~= 0  OutDataTypeStr=Inherit: Inherit via back propagation
  inv Lookup Table : Lookup_n-D  NumberOfTableDimensions=1  BreakpointsForDimension1=frac_lut_table_breaks_coarse_cfo  IndexSearchMethod=Evenly spaced points  Table=frac_lut_table_data_coarse_cfo  InterpMethod=Flat  DiagnosticForOutOfRangeInput=Error  RemoveProtectionInput=on  InternalRulePriority=Speed  OutDataTypeStr=Inherit: Inherit via back propagation  RndMeth=Simplest  InputSameDT=on
  mult_delay : Delay  DelayLength=cr_mult_pipeline*2
  mult_delay_match : Delay  DelayLength=cr_mult_pipeline*2
  mult_delay_match1 : Delay  DelayLength=cr_mult_pipeline*2
  pipeline_delay1 : Delay  DelayLength=regular_pipeline
  pipeline_delay2 : Delay  DelayLength=regular_pipeline  InitialCondition=1
  pipeline_delay_match : Delay  DelayLength=regular_pipeline*2
  pipeline_delay_match1 : Delay  DelayLength=regular_pipeline*2
  Out : Outport  VectorParamsAs1DForOutWhenUnconnected=off
  wires:
  pipeline_delay2/1 -> Data Type Duplicate2/1, Switch2/3
  mult_delay/1 -> inv Lookup Table/1
  pipeline_delay1/1 -> mult_delay/1
  mult_delay_match1/1 -> Switch3/2
  mult_delay_match/1 -> Switch2/2
  pipeline_delay_match1/1 -> mult_delay_match1/1
  pipeline_delay_match/1 -> mult_delay_match/1
  inv Lookup Table/1 -> Data Type Duplicate/2, pipeline_delay2/1
  Switch8/1 -> Data Type Conversion/1
  Constant11/1 -> Switch8/1
  Logical Operator/1 -> Switch8/2
  Switch3/1 -> Data Type Duplicate2/2, Data Type Duplicate1/2, Out/1
  Constant4/1 -> Switch3/1
  Switch2/1 -> Data Type Duplicate1/1, Switch3/3
  Constant3/1 -> Switch2/1
  Compare To Constant4/1 -> pipeline_delay_match1/1, Logical Operator/2
  Compare To Constant1/1 -> pipeline_delay_match/1, Logical Operator/1
  In/1 -> Data Type Duplicate/1, Compare To Constant4/1, Compare To Constant1/1, Switch8/3
  Data Type Conversion/1 -> pipeline_delay1/1

== system cyclopsLib/cyclops_rx_combined/slow_rx_encapsulated/slow_rx/slow_rx_baseband_outer/slow_rx_baseband_enabled/slow_rx_baseband/FineCarrierRecovery/Est_Phase/atan2 ==
  note: 4 delays
  note: Special case for undefined ouput of atan2.
      | To produce an unbiased ouput, this should be 0.
  imag_y : Inport
  real_x : Inport  Port=2
  Add : Sum
  Compare To Constant1 : simulink/Logic and Bit Operations/Compare To Constant  relop=>=  const=0  OutDataTypeStr=boolean
  Compare To Constant2 : simulink/Logic and Bit Operations/Compare To Constant  relop=>=  const=0  OutDataTypeStr=boolean
  Compare To Constant3 : simulink/Logic and Bit Operations/Compare To Constant  relop===  const=0  OutDataTypeStr=boolean
  Compare To Constant4 : simulink/Logic and Bit Operations/Compare To Constant  relop===  const=0  OutDataTypeStr=boolean
  Constant : Constant  Value=pi  OutDataTypeStr=Inherit: Inherit via back propagation  SampleTime=-1
  Constant2 : Constant  Value=0  OutDataTypeStr=Inherit: Inherit via back propagation  SampleTime=-1
  Constant3 : Constant  Value=-pi/2  OutDataTypeStr=Inherit: Inherit via back propagation  SampleTime=-1
  Constant4 : Constant  Value=pi/2  OutDataTypeStr=Inherit: Inherit via back propagation  SampleTime=-1
  Logical Operator : Logic  AllPortsSameDT=off  OutDataTypeStr=boolean
  Logical Operator1 : Logic  AllPortsSameDT=off  OutDataTypeStr=boolean
  Sub : Sum  Inputs=+-
  Switch{1,3..5,8} (5 alike) : Switch  Criteria=u2 ~= 0  OutDataTypeStr=Inherit: Inherit via back propagation
  bound_atan : Subsystem  AncestorBlock=helperLib/bound_atan
  inv : Subsystem
  mult_delay_match : Delay  DelayLength=cr_mult_pipeline*2+regular_pipeline*2
  pipeline_delay{,1..3} (4 alike) : Delay  DelayLength=regular_pipeline
  pipeline_delay_match{,1..4} (5 alike) : Delay  DelayLength=cr_mult_pipeline*5+regular_pipeline*7
  pipelined_mult : helperLib/pipelined_mult  d=cr_mult_pipeline
  Out1 : Outport  VectorParamsAs1DForOutWhenUnconnected=off
  wires:
  pipeline_delay1/1 -> bound_atan/1(In1)
  pipeline_delay_match/1 -> Switch1/2
  pipeline_delay_match1/1 -> Switch8/2
  imag_y/1 -> Compare To Constant4/1, Compare To Constant2/1, mult_delay_match/1
  Sub/1 -> Switch1/3
  Constant/1 -> Sub/2, Add/2
  Add/1 -> Switch1/1
  Switch1/1 -> Switch8/3
  Compare To Constant2/1 -> Logical Operator1/1, pipeline_delay_match/1
  Compare To Constant1/1 -> pipeline_delay_match1/1
  pipeline_delay/1 -> Sub/1, Add/1, Switch8/1
  mult_delay_match/1 -> pipeline_delay2/1
  bound_atan/1(Out1) -> pipeline_delay/1
  pipelined_mult/1 -> pipeline_delay1/1
  pipeline_delay2/1 -> pipelined_mult/1
  pipeline_delay3/1 -> pipelined_mult/2
  Compare To Constant4/1 -> Logical Operator/1
  Logical Operator/1 -> pipeline_delay_match2/1
  pipeline_delay_match2/1 -> Switch3/2
  real_x/1 -> inv/1(In), Compare To Constant3/1, Compare To Constant1/1
  inv/1(Out) -> pipeline_delay3/1
  Switch8/1 -> Switch4/3
  Switch4/1 -> Switch5/3
  Constant3/1 -> Switch4/1
  Constant4/1 -> Switch5/1
  Switch5/1 -> Switch3/3
  Constant2/1 -> Switch3/1
  Switch3/1 -> Out1/1
  Compare To Constant3/1 -> Logical Operator1/2, pipeline_delay_match4/1, Logical Operator/2
  Logical Operator1/1 -> pipeline_delay_match3/1
  pipeline_delay_match3/1 -> Switch5/2
  pipeline_delay_match4/1 -> Switch4/2

== system cyclopsLib/cyclops_rx_combined/slow_rx_encapsulated/slow_rx/slow_rx_baseband_outer/slow_rx_baseband_enabled/slow_rx_baseband/FineCarrierRecovery/Est_Phase/complex_mult_pipelined1 ==
  In1 : Inport
  In2 : Inport  Port=2
  Add1 : Sum  OutDataTypeStr=Inherit: Same as first input
  Add2 : Sum  OutDataTypeStr=Inherit: Same as first input
  Complex to Real-Imag3 : ComplexToRealImag
  Complex to Real-Imag4 : ComplexToRealImag
  Real-Imag to Complex2 : RealImagToComplex
  mult_delay_match3 : Delay  DelayLength=cr_mult_pipeline
  mult_delay_match4 : Delay  DelayLength=cr_mult_pipeline
  mult_delay_match5 : Delay  DelayLength=cr_mult_pipeline
  pipeline_delay{1..3,6} (4 alike) : Delay  DelayLength=regular_pipeline
  pipelined_gain : helperLib/pipelined_gain  g=-1  d=cr_mult_pipeline
  pipelined_mult{,1..3} (4 alike) : helperLib/pipelined_mult  d=cr_mult_pipeline
  Out1 : Outport  VectorParamsAs1DForOutWhenUnconnected=off
  wires:
  pipelined_gain/1 -> Add1/2
  pipelined_mult3/1 -> mult_delay_match5/1
  pipelined_mult2/1 -> mult_delay_match4/1
  pipelined_mult1/1 -> pipelined_gain/1
  pipelined_mult/1 -> mult_delay_match3/1
  Complex to Real-Imag4/1 -> pipelined_mult/2, pipelined_mult3/2
  Complex to Real-Imag3/2 -> pipelined_mult1/1, pipelined_mult3/1
  Complex to Real-Imag4/2 -> pipelined_mult2/2, pipelined_mult1/2
  Complex to Real-Imag3/1 -> pipelined_mult2/1, pipelined_mult/1
  pipeline_delay3/1 -> Complex to Real-Imag4/1
  pipeline_delay2/1 -> Complex to Real-Imag3/1
  Add2/1 -> pipeline_delay6/1
  Add1/1 -> pipeline_delay1/1
  In1/1 -> pipeline_delay2/1
  mult_delay_match5/1 -> Add2/2
  pipeline_delay1/1 -> Real-Imag to Complex2/1
  In2/1 -> pipeline_delay3/1
  pipeline_delay6/1 -> Real-Imag to Complex2/2
  Real-Imag to Complex2/1 -> Out1/1
  mult_delay_match3/1 -> Add1/1
  mult_delay_match4/1 -> Add2/1

== system cyclopsLib/cyclops_rx_combined/slow_rx_encapsulated/slow_rx/slow_rx_baseband_outer/slow_rx_baseband_enabled/slow_rx_baseband/FineCarrierRecovery/Est_Phase/find_nearest ==
  In1 : Inport
  ModMode : Inport  Port=2
  BPSK Demodulator Baseband : commdigbbndpm3/BPSK Demodulator Baseband  DecType=Hard decision  VarSource=Dialog  Variance=1  Ph=0  outDtype=boolean  derotateFactorWordLen=16  derotateFactorDataTypeStr=Inherit: Same word length as input  derotateFactorLastDataTypeStr=Inherit: Same word length as input
  BPSK Modulator Baseband : commdigbbndpm3/BPSK Modulator Baseband  Ph=0  outDtype=single  outWordLen=25  outUDDataType=sfix(16)  outFracLenMode=User-defined  outFracLen=17  outDataTypeStr=single  outLastDataTypeStr=single
  Gain : Gain  Gain=qam16_demod_scale_factor
  Multiport Switch : MultiPortSwitch
  QPSK Demodulator Baseband : commdigbbndpm3/QPSK Demodulator Baseband  OutType=Integer  DecType=Hard decision  VarSource=Dialog  Variance=1  Dec=Gray  Ph=pi/4  outDtype1=Inherit via internal rule  outDtype2=uint8  derotateFactorWordLen=16  derotateFactorDataTypeStr=Inherit: Same word length as input  derotateFactorLastDataTypeStr=Inherit: Same word length as input
  QPSK Modulator Baseband : commdigbbndpm3/QPSK Modulator Baseband  InType=Integer  Enc=Gray  Ph=pi/4  outDtype=single  outWordLen=25  outUDDataType=sfix(16)  outFracLenMode=User-defined  outFracLen=17  outDataTypeStr=single  outLastDataTypeStr=single
  Rectangular QAM Demodulator Baseband1 : commdigbbndam3/Rectangular QAM Demodulator Baseband  M=16  OutType=Integer  DecType=Hard decision  VarSource=Dialog  Variance=1  Dec=Gray  Mapping=[0:15]  PowType=Min. distance between symbols  MinDist=qam16_hdl_distance  AvgPow=1  PeakPow=1  Ph=0  outDtype1=Inherit via internal rule  outDtype2=uint8  derotateFactorWordLen=16  derotateFactorDataTypeStr=Inherit: Same word length as input  derotateFactorLastDataTypeStr=Inherit: Same word length as input  denormFactorWordLen=16  denormFactorDataTypeStr=Inherit: Same word length as input  denormFactorLastDataTypeStr=Inherit: Same word length as input  prodOutWordLen=32  prodOutOverflowMode=Wrap  prodOutRoundingMode=Floor  prodOutOvFlMode=off  prodOutOvFlModeLastStrValue=off  sumWordLen=32
  Rectangular QAM Modulator Baseband : commdigbbndam3/Rectangular QAM Modulator Baseband  M=16  InType=Integer  Enc=Gray  Mapping=[0:15]  PowType=Average Power  MinDist=2  AvgPow=1  PeakPow=1  Ph=0  outDtype=single  outWordLen=25  outUDDataType=sfix(16)  outFracLenMode=User-defined  outFracLen=17  outDataTypeStr=single  outLastDataTypeStr=single
  Out1 : Outport  VectorParamsAs1DForOutWhenUnconnected=off
  wires:
  BPSK Demodulator Baseband/1 -> BPSK Modulator Baseband/1
  In1/1 -> Gain/1, QPSK Demodulator Baseband/1, BPSK Demodulator Baseband/1
  QPSK Demodulator Baseband/1 -> QPSK Modulator Baseband/1
  Multiport Switch/1 -> Out1/1
  BPSK Modulator Baseband/1 -> Multiport Switch/2
  QPSK Modulator Baseband/1 -> Multiport Switch/3
  Rectangular QAM Modulator Baseband/1 -> Multiport Switch/4
  ModMode/1 -> Multiport Switch/1
  Gain/1 -> Rectangular QAM Demodulator Baseband1/1
  Rectangular QAM Demodulator Baseband1/1 -> Rectangular QAM Modulator Baseband/1

== system cyclopsLib/cyclops_rx_combined/slow_rx_encapsulated/slow_rx/slow_rx_baseband_outer/slow_rx_baseband_enabled/slow_rx_baseband/FineCarrierRecovery/scale_and_loop/Loop Filter ==
  PhaseOffset : Inport
  cr_i_preamp : Inport  Port=2
  cr_p : Inport  Port=3
  cr_i : Inport  Port=4
  cr_integrator1_decay : Inport  Port=5
  cr_int1_sat_up : Inport  Port=6
  cr_int1_sat_low : Inport  Port=7
  cr_sat2_up : Inport  Port=8
  cr_sat2_low : Inport  Port=9
  int1_freeze : Inport  Port=10  OutDataTypeStr=boolean
  reset : Inport  Port=11
  Add1 : Sum  OutDataTypeStr=Inherit: Same as first input
  Add2 : Sum  OutDataTypeStr=Inherit: Same as first input
  Constant : Constant  Value=0  OutDataTypeStr=Inherit: Inherit via back propagation  SampleTime=-1
  Constant1 : Constant  Value=0  OutDataTypeStr=Inherit: Inherit via back propagation  SampleTime=-1
  Data Type Duplicate{1..3,5} (4 alike) : DataTypeDuplicate
  Delay1 : Delay  DelayLength=1  InitialCondition=0
  Discrete FIR Filter : DiscreteFir  FilterStructure=Direct form transposed  Coefficients=cr_smooth_num  OutDataTypeStr=Inherit: Same as input
  Switch1 : Switch  Criteria=u2 > Threshold
  Switch2 : Switch  Criteria=u2 > Threshold
  Switch3 : Switch  Criteria=u2 > Threshold
  cr_components : Scope  NumInputPorts=2
  pipeline_delay{3..8} (6 alike) : Delay  DelayLength=regular_pipeline
  pipelined_mult{,1..2,4} (4 alike) : helperLib/pipelined_mult  d=cr_mult_pipeline
  sat : Subsystem
  sat2 : Subsystem
  Out : Outport  VectorParamsAs1DForOutWhenUnconnected=off
  wires:
  Add1/1 -> sat/1(In1)
  Switch2/1 -> Add2/1
  pipeline_delay5/1 -> Add1/1
  PhaseOffset/1 -> pipeline_delay8/1
  sat/1(Out1) -> pipelined_mult2/1, Switch3/3, Data Type Duplicate3/1
  cr_p/1 -> pipelined_mult/2, Data Type Duplicate2/2
  Discrete FIR Filter/1 -> Data Type Duplicate2/1, pipelined_mult/1, Data Type Duplicate1/1, pipelined_mult1/1
  cr_i_preamp/1 -> pipelined_mult1/2, Data Type Duplicate1/2
  pipelined_mult1/1 -> pipeline_delay5/1
  cr_i/1 -> pipelined_mult2/2, Data Type Duplicate3/2
  pipelined_mult2/1 -> pipeline_delay4/1
  cr_integrator1_decay/1 -> Data Type Duplicate5/2, pipelined_mult4/2
  pipelined_mult/1 -> pipeline_delay3/1
  cr_int1_sat_up/1 -> sat/2(limit_up)
  cr_int1_sat_low/1 -> sat/3(limit_low)
  cr_sat2_up/1 -> sat2/2(limit_up)
  cr_sat2_low/1 -> sat2/3(limit_low)
  Delay1/1 -> Switch1/1
  int1_freeze/1 -> Switch2/2, Switch1/2
  Switch1/1 -> Delay1/1, Add2/2
  pipeline_delay4/1 -> cr_components/2, Switch1/3
  pipeline_delay3/1 -> cr_components/1, Switch2/3
  Constant/1 -> Switch2/1
  pipeline_delay8/1 -> Discrete FIR Filter/1
  pipeline_delay7/1 -> sat2/1(In1)
  sat2/1(Out1) -> pipeline_delay6/1
  pipeline_delay6/1 -> Out/1
  Add2/1 -> pipeline_delay7/1
  Constant1/1 -> Switch3/1
  reset/1 -> Switch3/2
  pipelined_mult4/1 -> Add1/2
  Switch3/1 -> Data Type Duplicate5/1, pipelined_mult4/1
